simulink model "Stateflow_Moore_example"  (R2014a)
settings: Solver=FixedStepDiscrete  StartTime=0.0  StopTime=10.0  RelTol=1e-3
settings Model: Creator=mprior  LastModifiedBy=mprior
settings DataIOCC: LimitDataPoints=off  SaveOutput=off  SaveTime=off
settings DebuggingCC: SolverPrmCheckMsg=none  SingleTaskRateTransMsg=error

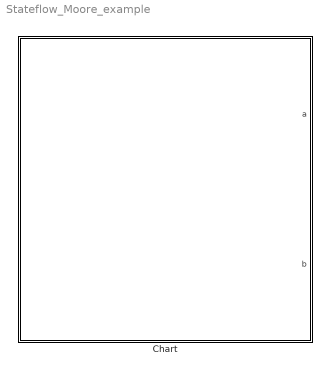
== system Stateflow_Moore_example ==
  Chart : Stateflow chart  TreatAsAtomicUnit=on

== stateflow chart Stateflow_Moore_example/Chart ==
  settings: stateMachineType=MOORE_MACHINE
  state INITIAL
    a=0; b=0
  state IDLE
    a=0;
  state FINAL
  state SEQ1
    a=1; b=b+1
  state SEQ2
  (default) -> INITIAL
  INITIAL -> IDLE
  FINAL -> IDLE
  IDLE -> SEQ1
  SEQ2 -> FINAL
  SEQ1 -> SEQ2
  data: a output double; b output double
